simulink library "InterpolationLib"  (R2020b)
settings: Solver=VariableStepAuto  StartTime=0.0  StopTime=10.0  RelTol=1e-3
Description:
  | VLS Standard Library
  | Version: 1.0.0
settings Model: Creator=mchawa  LastModifiedBy=ahashem
settings DataIOCC: ReturnWorkspaceOutputs=off
settings DebuggingCC: ArithmeticOperatorsInVariantConditions=warning
settings SFSimCC: SimUseLocalCustomCode=off  CustomCodeUndefinedFunction=UseInterfaceOnly
settings RTWCC: RTWUseLocalCustomCode=off

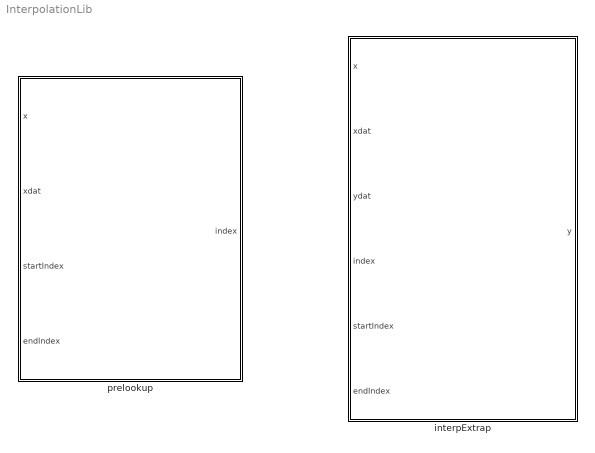
== system InterpolationLib ==
  interpExtrap : Subsystem
  prelookup : Subsystem  TreatAsAtomicUnit=on

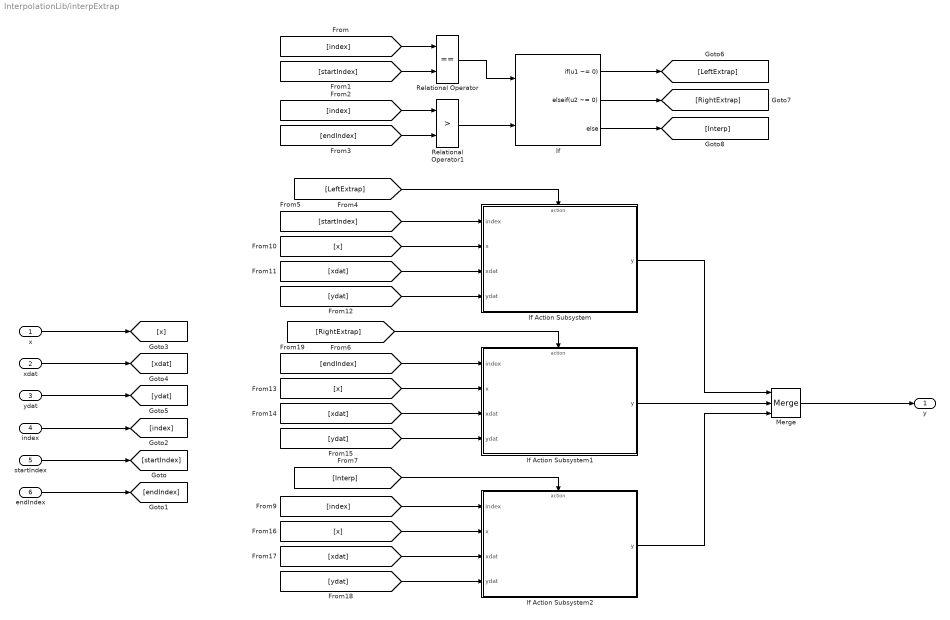
== system InterpolationLib/interpExtrap ==
  x : Inport
  xdat : Inport  Port=2
  ydat : Inport  Port=3
  index : Inport  Port=4
  startIndex : Inport  Port=5
  endIndex : Inport  Port=6
  If : If  NumInputs=2  IfExpression=u1 ~= 0  ElseIfExpressions=u2 ~= 0
  If Action Subsystem : Subsystem  TreatAsAtomicUnit=on
  If Action Subsystem1 : Subsystem  TreatAsAtomicUnit=on
  If Action Subsystem2 : Subsystem  TreatAsAtomicUnit=on
  Merge : Merge  Inputs=3
  Relational Operator : RelationalOperator  Operator===  OutDataTypeStr=boolean  RndMeth=Simplest
  Relational Operator1 : RelationalOperator  Operator=>  OutDataTypeStr=boolean  RndMeth=Simplest
  y : Outport  VectorParamsAs1DForOutWhenUnconnected=off
  wires:
  startIndex/1 -> [startIndex]
  endIndex/1 -> [endIndex]
  index/1 -> [index]
  x/1 -> [x]
  xdat/1 -> [xdat]
  ydat/1 -> [ydat]
  Relational Operator/1 -> If/1
  Relational Operator1/1 -> If/2
  [index] -> Relational Operator/1
  [startIndex] -> Relational Operator/2
  [index] -> Relational Operator1/1
  [endIndex] -> Relational Operator1/2
  If/1 -> [LeftExtrap]
  If/2 -> [RightExtrap]
  If/3 -> [Interp]
  [LeftExtrap] -> If Action Subsystem/Action
  [RightExtrap] -> If Action Subsystem1/Action
  [Interp] -> If Action Subsystem2/Action
  [endIndex] -> If Action Subsystem1/1(index)
  [index] -> If Action Subsystem2/1(index)
  [x] -> If Action Subsystem/2(x)
  [xdat] -> If Action Subsystem/3(xdat)
  [ydat] -> If Action Subsystem/4(ydat)
  [x] -> If Action Subsystem1/2(x)
  [xdat] -> If Action Subsystem1/3(xdat)
  [ydat] -> If Action Subsystem1/4(ydat)
  [x] -> If Action Subsystem2/2(x)
  [xdat] -> If Action Subsystem2/3(xdat)
  [ydat] -> If Action Subsystem2/4(ydat)
  If Action Subsystem1/1(y) -> Merge/2
  If Action Subsystem/1(y) -> Merge/1
  If Action Subsystem2/1(y) -> Merge/3
  Merge/1 -> y/1
  [startIndex] -> If Action Subsystem/1(index)

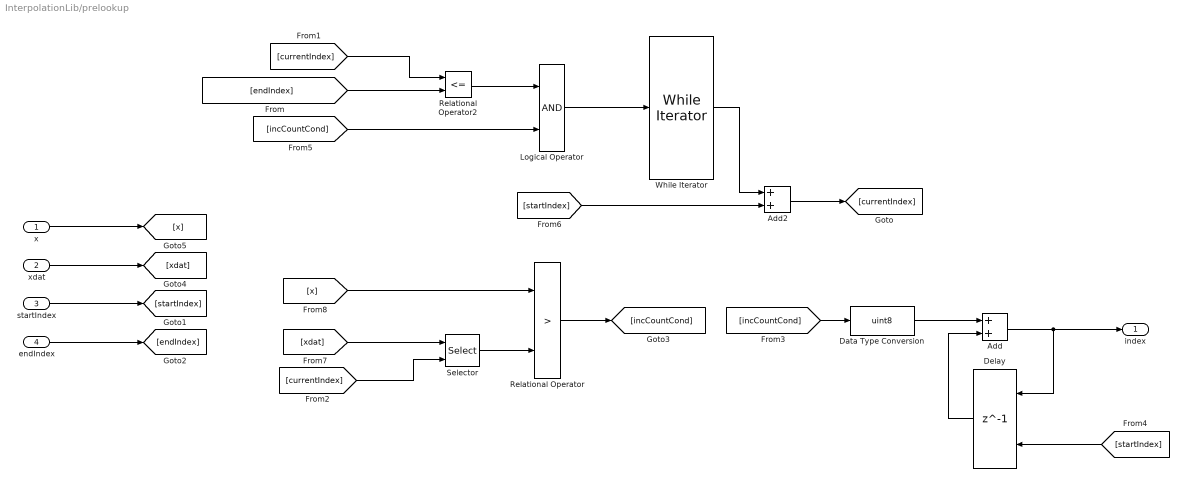
== system InterpolationLib/prelookup ==
  x : Inport
  xdat : Inport  Port=2
  startIndex : Inport  Port=3
  endIndex : Inport  Port=4
  Add : Sum
  Add2 : Sum
  Data Type Conversion : DataTypeConversion  OutDataTypeStr=uint8
  Delay : Delay  DelayLength=1  InitialConditionSource=Input port
      settings: InputPortMap=u0,p4
  Logical Operator : Logic  AllPortsSameDT=off  OutDataTypeStr=boolean
  Relational Operator : RelationalOperator  Operator=>  OutDataTypeStr=boolean  RndMeth=Simplest
  Relational Operator2 : RelationalOperator  Operator=<=  OutDataTypeStr=boolean  RndMeth=Simplest
  Selector : Selector  IndexOptions=Index vector (port)  Indices=[1 3]  OutputSizes=1
  While Iterator : WhileIterator  MaxIters=-1  WhileBlockType=do-while  ResetStates=reset  ShowIterationPort=on
  index : Outport  VectorParamsAs1DForOutWhenUnconnected=off
  wires:
  Add/1 -> Delay/1, index/1
  Data Type Conversion/1 -> Add/1
  Selector/1 -> Relational Operator/2
  [currentIndex] -> Selector/2
  startIndex/1 -> [startIndex]
  While Iterator/1 -> Add2/1
  Add2/1 -> [currentIndex]
  [startIndex] -> Add2/2
  endIndex/1 -> [endIndex]
  [endIndex] -> Relational Operator2/2
  Logical Operator/1 -> While Iterator/1
  Relational Operator2/1 -> Logical Operator/1
  Relational Operator/1 -> [incCountCond]
  [incCountCond] -> Data Type Conversion/1
  Delay/1 -> Add/2
  [startIndex] -> Delay/2
  xdat/1 -> [xdat]
  [xdat] -> Selector/1
  x/1 -> [x]
  [x] -> Relational Operator/1
  [incCountCond] -> Logical Operator/2
  [currentIndex] -> Relational Operator2/1

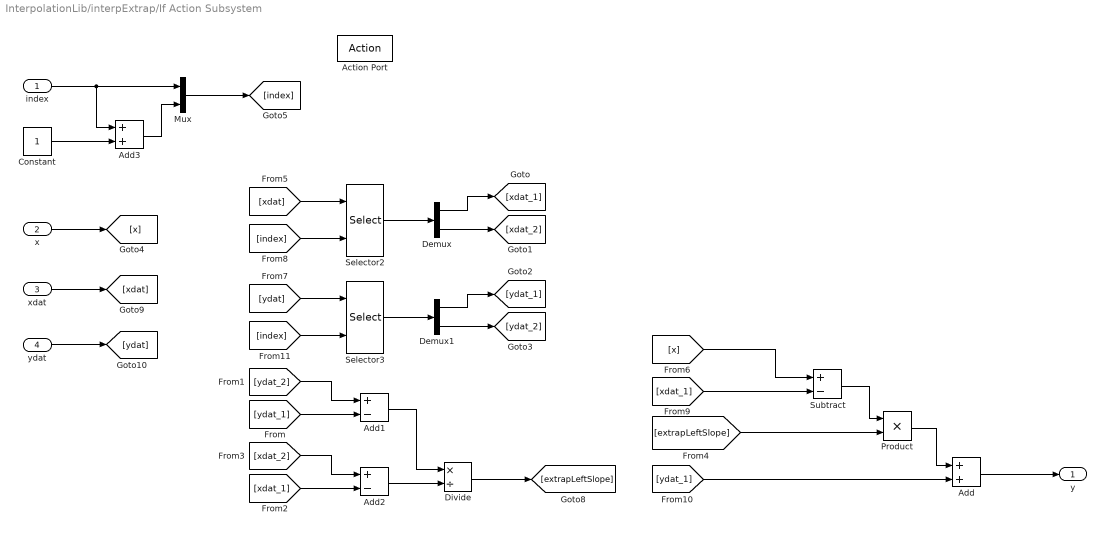
== system InterpolationLib/interpExtrap/If Action Subsystem ==
  index : Inport
  x : Inport  Port=2
  xdat : Inport  Port=3
  ydat : Inport  Port=4
  Action Port : ActionPort
  Add : Sum  SaturateOnIntegerOverflow=on
  Add1 : Sum  Inputs=+-  OutDataTypeStr=fixdt(1,16,0.1,0)
  Add2 : Sum  Inputs=+-  OutDataTypeStr=fixdt(1,16,0.1,0)
  Add3 : Sum
  Constant : Constant  OutDataTypeStr=uint8
  Demux : Demux  Outputs=2
  Demux1 : Demux  Outputs=2
  Divide : Product  Inputs=*/  OutDataTypeStr=fixdt(1,32,0.0001,0)
  Mux : Mux  Inputs=2
  Product : Product  OutDataTypeStr=fixdt(1,32,0.00001,0)
  Selector2 : Selector  IndexMode=Zero-based  IndexOptions=Index vector (port)  Indices=[1 2]  OutputSizes=1
  Selector3 : Selector  IndexMode=Zero-based  IndexOptions=Index vector (port)  Indices=[1 2]  OutputSizes=1
  Subtract : Sum  Inputs=+-
  y : Outport  VectorParamsAs1DForOutWhenUnconnected=off
  wires:
  ydat/1 -> [ydat]
  xdat/1 -> [xdat]
  [xdat] -> Selector2/1
  Selector2/1 -> Demux/1
  Demux1/2 -> [ydat_2]
  [ydat] -> Selector3/1
  Demux1/1 -> [ydat_1]
  Demux/2 -> [xdat_2]
  Selector3/1 -> Demux1/1
  [xdat_1] -> Subtract/2
  Product/1 -> Add/1
  Subtract/1 -> Product/1
  [ydat_1] -> Add/2
  Add2/1 -> Divide/2
  Demux/1 -> [xdat_1]
  Divide/1 -> [extrapLeftSlope]
  Add/1 -> y/1
  [extrapLeftSlope] -> Product/2
  Add1/1 -> Divide/1
  x/1 -> [x]
  [x] -> Subtract/1
  index/1 -> Mux/1, Add3/1
  Add3/1 -> Mux/2
  Constant/1 -> Add3/2
  Mux/1 -> [index]
  [index] -> Selector2/2
  [index] -> Selector3/2
  [ydat_1] -> Add1/2
  [ydat_2] -> Add1/1
  [xdat_1] -> Add2/2
  [xdat_2] -> Add2/1

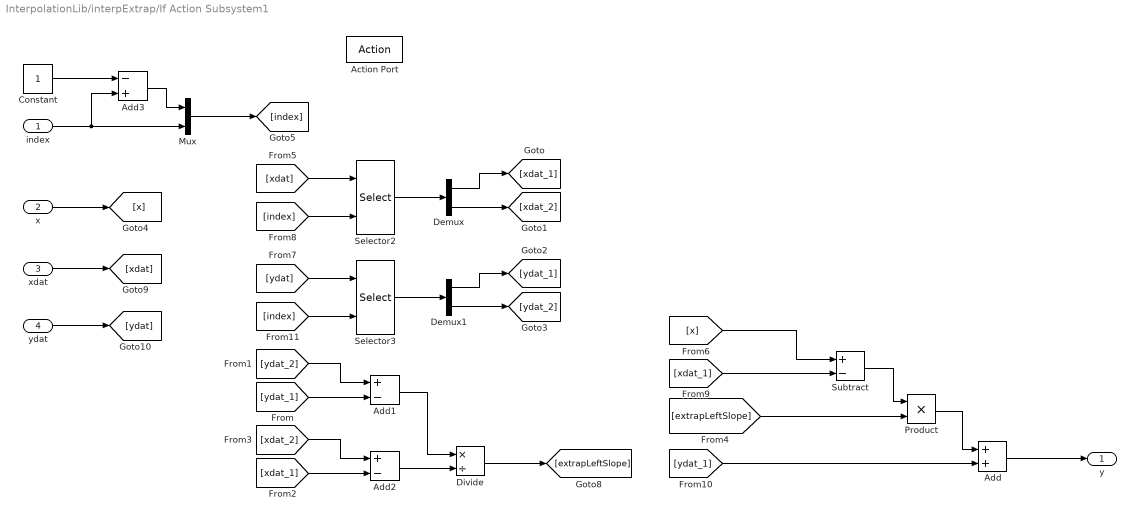
== system InterpolationLib/interpExtrap/If Action Subsystem1 ==
  index : Inport
  x : Inport  Port=2
  xdat : Inport  Port=3
  ydat : Inport  Port=4
  Action Port : ActionPort
  Add : Sum  SaturateOnIntegerOverflow=on
  Add1 : Sum  Inputs=+-  OutDataTypeStr=fixdt(1,16,0.1,0)
  Add2 : Sum  Inputs=+-  OutDataTypeStr=fixdt(1,16,0.1,0)
  Add3 : Sum  Inputs=-+
  Constant : Constant  OutDataTypeStr=uint8
  Demux : Demux  Outputs=2
  Demux1 : Demux  Outputs=2
  Divide : Product  Inputs=*/  OutDataTypeStr=fixdt(1,32,0.0001,0)
  Mux : Mux  Inputs=2
  Product : Product  OutDataTypeStr=fixdt(1,32,0.00001,0)
  Selector2 : Selector  IndexMode=Zero-based  IndexOptions=Index vector (port)  Indices=[1 2]  OutputSizes=1
  Selector3 : Selector  IndexMode=Zero-based  IndexOptions=Index vector (port)  Indices=[1 2]  OutputSizes=1
  Subtract : Sum  Inputs=+-
  y : Outport  VectorParamsAs1DForOutWhenUnconnected=off
  wires:
  [index] -> Selector3/2
  [index] -> Selector2/2
  Mux/1 -> [index]
  Constant/1 -> Add3/1
  [x] -> Subtract/1
  x/1 -> [x]
  Add1/1 -> Divide/1
  [extrapLeftSlope] -> Product/2
  Add/1 -> y/1
  Divide/1 -> [extrapLeftSlope]
  Demux/1 -> [xdat_1]
  Add2/1 -> Divide/2
  [ydat_1] -> Add/2
  Subtract/1 -> Product/1
  Product/1 -> Add/1
  [xdat_1] -> Subtract/2
  Selector3/1 -> Demux1/1
  Demux/2 -> [xdat_2]
  Demux1/1 -> [ydat_1]
  [ydat] -> Selector3/1
  Demux1/2 -> [ydat_2]
  Selector2/1 -> Demux/1
  [xdat] -> Selector2/1
  xdat/1 -> [xdat]
  ydat/1 -> [ydat]
  index/1 -> Add3/2, Mux/2
  Add3/1 -> Mux/1
  [ydat_1] -> Add1/2
  [ydat_2] -> Add1/1
  [xdat_1] -> Add2/2
  [xdat_2] -> Add2/1

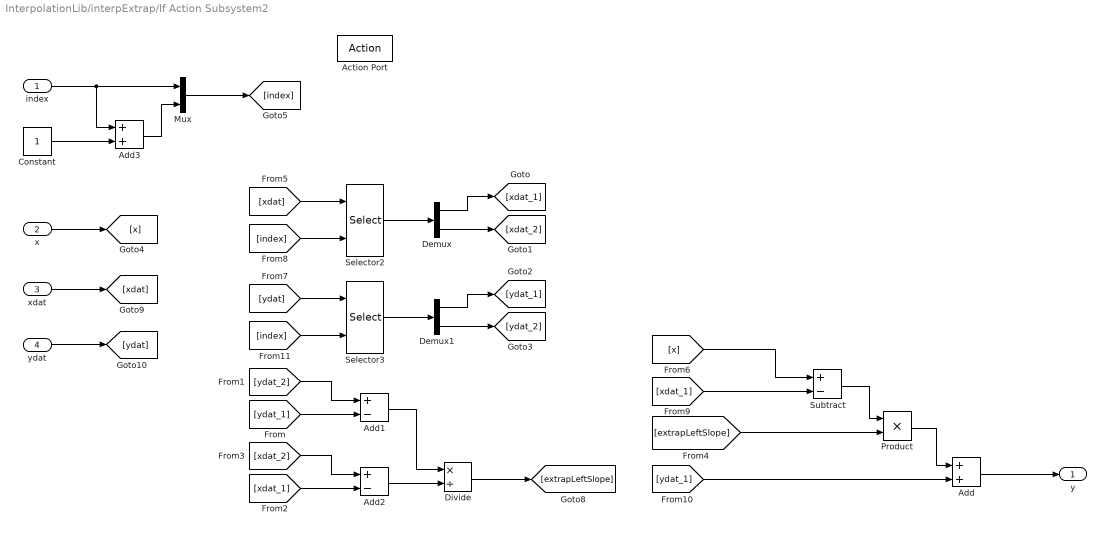
== system InterpolationLib/interpExtrap/If Action Subsystem2 ==
  index : Inport
  x : Inport  Port=2
  xdat : Inport  Port=3
  ydat : Inport  Port=4
  Action Port : ActionPort
  Add : Sum  SaturateOnIntegerOverflow=on
  Add1 : Sum  Inputs=+-  OutDataTypeStr=fixdt(1,16,0.1,0)
  Add2 : Sum  Inputs=+-  OutDataTypeStr=fixdt(1,16,0.1,0)
  Add3 : Sum
  Constant : Constant  OutDataTypeStr=uint8
  Demux : Demux  Outputs=2
  Demux1 : Demux  Outputs=2
  Divide : Product  Inputs=*/  OutDataTypeStr=fixdt(1,32,0.0001,0)
  Mux : Mux  Inputs=2
  Product : Product  OutDataTypeStr=fixdt(1,32,0.00001,0)
  Selector2 : Selector  IndexOptions=Index vector (port)  Indices=[1 2]  OutputSizes=1
  Selector3 : Selector  IndexOptions=Index vector (port)  Indices=[1 2]  OutputSizes=1
  Subtract : Sum  Inputs=+-
  y : Outport  VectorParamsAs1DForOutWhenUnconnected=off
  wires:
  [xdat_2] -> Add2/1
  [xdat_1] -> Add2/2
  [ydat_2] -> Add1/1
  [ydat_1] -> Add1/2
  [index] -> Selector3/2
  [index] -> Selector2/2
  Mux/1 -> [index]
  Constant/1 -> Add3/2
  Add3/1 -> Mux/2
  index/1 -> Add3/1, Mux/1
  [x] -> Subtract/1
  x/1 -> [x]
  Add1/1 -> Divide/1
  [extrapLeftSlope] -> Product/2
  Add/1 -> y/1
  Divide/1 -> [extrapLeftSlope]
  Demux/1 -> [xdat_1]
  Add2/1 -> Divide/2
  [ydat_1] -> Add/2
  Subtract/1 -> Product/1
  Product/1 -> Add/1
  [xdat_1] -> Subtract/2
  Selector3/1 -> Demux1/1
  Demux/2 -> [xdat_2]
  Demux1/1 -> [ydat_1]
  [ydat] -> Selector3/1
  Demux1/2 -> [ydat_2]
  Selector2/1 -> Demux/1
  [xdat] -> Selector2/1
  xdat/1 -> [xdat]
  ydat/1 -> [ydat]
